simulink model "NeuromuscularModel_3R60CMG_3D"  (R2019b)
settings: Solver=ode15s  StartTime=0.0  StopTime=20  MaxStep=.001  MinStep=1e-34  RelTol=1e-5  AbsTol=1e-7  EnableMultiTasking=on
values from neighbouring files (symbols this model uses):
  animFrameRate = 30    [demorun.m]    (also in evaluateCost.m; optimize.m; optimizeCMG.m)
  dt_visual = 1/1000    (= 0.001)    [demorun.m]    (also in evaluateCost.m; optimize.m = 0.0333333333333; optimizeCMG.m)
  initialTargetAngle = 70*pi/180    (= 1.2217304764)    [setInit.m]
  LPreStimBFSHinit = initConditionsSagittal(12)    [assignInit.m]
  LPreStimGASinit = initConditionsSagittal(13)    [assignInit.m]
  LPreStimGLUinit = initConditionsSagittal(8)    [assignInit.m]
  LPreStimHABinit = initConditionsCoronal(6)    [assignInit.m]
  LPreStimHADinit = initConditionsCoronal(7)    [assignInit.m]
  LPreStimHAMinit = initConditionsSagittal(9)    [assignInit.m]
  LPreStimHFLinit = initConditionsSagittal(7)    [assignInit.m]
  LPreStimRFinit = initConditionsSagittal(10)    [assignInit.m]
  LPreStimSOLinit = initConditionsSagittal(14)    [assignInit.m]
  LPreStimTAinit = initConditionsSagittal(15)    [assignInit.m]
  LPreStimVASinit = initConditionsSagittal(11)    [assignInit.m]
  LTargetAngleInit = initConditionsSagittal(6)    [assignInit.m]
  LTargetAngleRInit = initConditionsCoronal(5)    [assignInit.m]
  RPreStimGLUinit = initConditionsSagittal(18)    [assignInit.m]
  RPreStimHABinit = initConditionsCoronal(9)    [assignInit.m]
  RPreStimHADinit = initConditionsCoronal(10)    [assignInit.m]
  RPreStimHAMinit = initConditionsSagittal(19)    [assignInit.m]
  RPreStimHFLinit = initConditionsSagittal(17)    [assignInit.m]
  RPreStimRFinit = initConditionsSagittal(20)    [assignInit.m]
  RTargetAngleInit = initConditionsSagittal(16)    [assignInit.m]
  RTargetAngleRInit = initConditionsCoronal(8)    [assignInit.m]
undefined symbols (not defined in the file or in its folder): DiscIntNeverNeededParam, g, hatLeftHipToCenterDistWidth, LongDelay, LongLoopDelay, MidDelay, ShortDelay, termination_height, thetaHATref, X, Y, Z
libraries: NeuroMuscularLibrary x96, nesl_utility x22, sm_lib x21, CMGlibrary x6, simulink x3
(part 3 of 3)

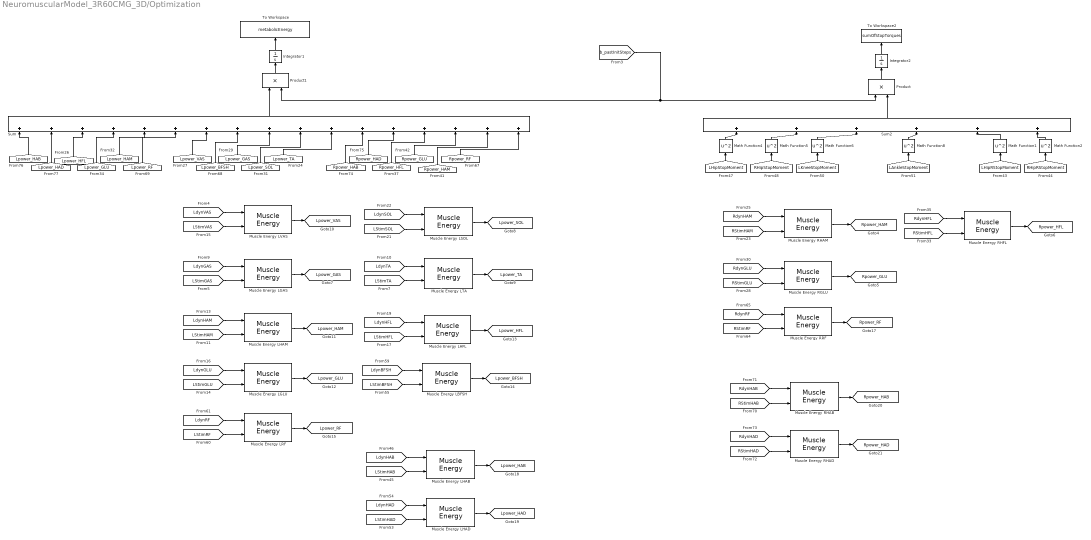
== system NeuromuscularModel_3R60CMG_3D/Optimization ==
  Integrator1 : Integrator
  Integrator2 : Integrator
  Math Function{1..2,4..6,8} (6 alike) : Math  Operator=square  SaturateOnIntegerOverflow=on
  Muscle Energy LBFSH : NeuroMuscularLibrary/Muscle Energy  lopt=loptBFSH  FT=FT_BFSH  Fmax=FmaxBFSH  vmax=vmaxBFSH
  Muscle Energy LGAS : NeuroMuscularLibrary/Muscle Energy  lopt=loptGAS  FT=FT_GAS  Fmax=FmaxGAS  vmax=vmaxGAS
  Muscle Energy LGLU : NeuroMuscularLibrary/Muscle Energy  lopt=loptGLU  FT=FT_GLU  Fmax=FmaxGLU  vmax=vmaxGLU
  Muscle Energy LHAB : NeuroMuscularLibrary/Muscle Energy  lopt=loptHAB  FT=FT_HAB  Fmax=FmaxHAB  vmax=vmaxHAB
  Muscle Energy LHAD : NeuroMuscularLibrary/Muscle Energy  lopt=loptHAD  FT=FT_HAD  Fmax=FmaxHAD  vmax=vmaxHAD
  Muscle Energy LHAM : NeuroMuscularLibrary/Muscle Energy  lopt=loptHAM  FT=FT_HAM  Fmax=FmaxHAM  vmax=vmaxHAM
  Muscle Energy LHFL : NeuroMuscularLibrary/Muscle Energy  lopt=loptHFL  FT=FT_HFL  Fmax=FmaxHFL  vmax=vmaxHFL
  Muscle Energy LRF : NeuroMuscularLibrary/Muscle Energy  lopt=loptRF  FT=FT_RF  Fmax=FmaxRF  vmax=vmaxRF
  Muscle Energy LSOL : NeuroMuscularLibrary/Muscle Energy  lopt=loptSOL  FT=FT_SOL  Fmax=FmaxSOL  vmax=vmaxSOL
  Muscle Energy LTA : NeuroMuscularLibrary/Muscle Energy  lopt=loptTA  FT=FT_TA  Fmax=FmaxTA  vmax=vmaxTA
  Muscle Energy LVAS : NeuroMuscularLibrary/Muscle Energy  lopt=loptVAS  FT=FT_VAS  Fmax=FmaxVAS  vmax=vmaxVAS
  Muscle Energy RGLU : NeuroMuscularLibrary/Muscle Energy  lopt=loptGLUamp  FT=FT_GLUamp  Fmax=FmaxGLUamp  vmax=vmaxGLUamp
  Muscle Energy RHAB : NeuroMuscularLibrary/Muscle Energy  lopt=loptHABamp  FT=FT_HABamp  Fmax=FmaxHABamp  vmax=vmaxHABamp
  Muscle Energy RHAD : NeuroMuscularLibrary/Muscle Energy  lopt=loptHADamp  FT=FT_HADamp  Fmax=FmaxHADamp  vmax=vmaxHADamp
  Muscle Energy RHAM : NeuroMuscularLibrary/Muscle Energy  lopt=loptHAMamp  FT=FT_HAMamp  Fmax=FmaxHAMamp  vmax=vmaxHAMamp
  Muscle Energy RHFL : NeuroMuscularLibrary/Muscle Energy  lopt=loptHFLamp  FT=FT_HFLamp  Fmax=FmaxHFLamp  vmax=vmaxHFLamp
  Muscle Energy RRF : NeuroMuscularLibrary/Muscle Energy  lopt=loptRFamp  FT=FT_RFamp  Fmax=FmaxRFamp  vmax=vmaxRFamp
  Product : Product
  Product1 : Product
  Sum : Sum  Inputs=+++++++++++++++++
  Sum2 : Sum  Inputs=++++++
  To Workspace : ToWorkspace  VariableName=metabolicEnergy  SampleTime=-1
      settings: MaxDataPoints=1
  To Workspace2 : ToWorkspace  VariableName=sumOfStopTorques  SampleTime=-1
      settings: MaxDataPoints=1
  tag scope: Lpower_BFSH=global, Lpower_GAS=global, Lpower_GLU=global, Lpower_HAB=global, Lpower_HAD=global, Lpower_HAM=global, Lpower_HFL=global, Lpower_RF=global, Lpower_SOL=global, Lpower_TA=global, Lpower_VAS=global, Rpower_GLU=global, Rpower_HAB=global, Rpower_HAD=global, Rpower_HAM=global, Rpower_HFL=global, Rpower_RF=global
  wires:
  [RdynHAM] -> Muscle Energy RHAM/1
  [RStimHAM] -> Muscle Energy RHAM/2
  [RdynGLU] -> Muscle Energy RGLU/1
  [RStimGLU] -> Muscle Energy RGLU/2
  [RdynHFL] -> Muscle Energy RHFL/1
  [RStimHFL] -> Muscle Energy RHFL/2
  Muscle Energy RHAM/1 -> [Rpower_HAM]
  Muscle Energy RGLU/1 -> [Rpower_GLU]
  Muscle Energy RHFL/1 -> [Rpower_HFL]
  [Lpower_HAB] -> Sum/1
  [Lpower_VAS] -> Sum/7
  [Lpower_RF] -> Sum/6
  [Lpower_HAM] -> Sum/5
  [Lpower_GLU] -> Sum/4
  [Lpower_HFL] -> Sum/3
  [Lpower_HAD] -> Sum/2
  [LdynSOL] -> Muscle Energy LSOL/1
  [LStimSOL] -> Muscle Energy LSOL/2
  [LStimVAS] -> Muscle Energy LVAS/2
  [LStimGAS] -> Muscle Energy LGAS/2
  Muscle Energy LVAS/1 -> [Lpower_VAS]
  Muscle Energy LGAS/1 -> [Lpower_GAS]
  Muscle Energy LSOL/1 -> [Lpower_SOL]
  Muscle Energy LTA/1 -> [Lpower_TA]
  [LdynTA] -> Muscle Energy LTA/1
  [LStimTA] -> Muscle Energy LTA/2
  [LdynHAM] -> Muscle Energy LHAM/1
  [LStimHAM] -> Muscle Energy LHAM/2
  [LdynGLU] -> Muscle Energy LGLU/1
  [LStimGLU] -> Muscle Energy LGLU/2
  [LdynHFL] -> Muscle Energy LHFL/1
  [LStimHFL] -> Muscle Energy LHFL/2
  Muscle Energy LHAM/1 -> [Lpower_HAM]
  Muscle Energy LGLU/1 -> [Lpower_GLU]
  Muscle Energy LHFL/1 -> [Lpower_HFL]
  [LdynGAS] -> Muscle Energy LGAS/1
  [LdynVAS] -> Muscle Energy LVAS/1
  [Lpower_SOL] -> Sum/10
  [Rpower_HAM] -> Sum/16
  [Rpower_GLU] -> Sum/15
  [Rpower_HFL] -> Sum/14
  [Rpower_HAD] -> Sum/13
  [Rpower_HAB] -> Sum/12
  [Lpower_TA] -> Sum/11
  Integrator1/1 -> To Workspace/1
  Sum/1 -> Product1/1
  Integrator2/1 -> To Workspace2/1
  Math Function4/1 -> Sum2/1
  [LHipStopMoment] -> Math Function4/1
  Math Function5/1 -> Sum2/2
  [RHipStopMoment] -> Math Function5/1
  Math Function6/1 -> Sum2/3
  [LKneeStopMoment] -> Math Function6/1
  [LAnkleStopMoment] -> Math Function8/1
  Math Function8/1 -> Sum2/4
  Product/1 -> Integrator2/1
  Sum2/1 -> Product/2
  Product1/1 -> Integrator1/1
  Muscle Energy LBFSH/1 -> [Lpower_BFSH]
  [LStimBFSH] -> Muscle Energy LBFSH/2
  [LdynBFSH] -> Muscle Energy LBFSH/1
  [LdynRF] -> Muscle Energy LRF/1
  [LStimRF] -> Muscle Energy LRF/2
  Muscle Energy LRF/1 -> [Lpower_RF]
  Muscle Energy RRF/1 -> [Rpower_RF]
  [RdynRF] -> Muscle Energy RRF/1
  [RStimRF] -> Muscle Energy RRF/2
  [Lpower_BFSH] -> Sum/8
  [Lpower_GAS] -> Sum/9
  [Rpower_RF] -> Sum/17
  Math Function1/1 -> Sum2/5
  [LHipRStopMoment] -> Math Function1/1
  [RHipRStopMoment] -> Math Function2/1
  Muscle Energy LHAB/1 -> [Lpower_HAB]
  [LStimHAB] -> Muscle Energy LHAB/2
  [LdynHAB] -> Muscle Energy LHAB/1
  [LdynHAD] -> Muscle Energy LHAD/1
  [LStimHAD] -> Muscle Energy LHAD/2
  Muscle Energy LHAD/1 -> [Lpower_HAD]
  Muscle Energy RHAD/1 -> [Rpower_HAD]
  [RStimHAD] -> Muscle Energy RHAD/2
  [RdynHAD] -> Muscle Energy RHAD/1
  [RdynHAB] -> Muscle Energy RHAB/1
  [RStimHAB] -> Muscle Energy RHAB/2
  Muscle Energy RHAB/1 -> [Rpower_HAB]
  Math Function2/1 -> Sum2/6
  [b_pastInitSteps] -> Product1/2, Product/1

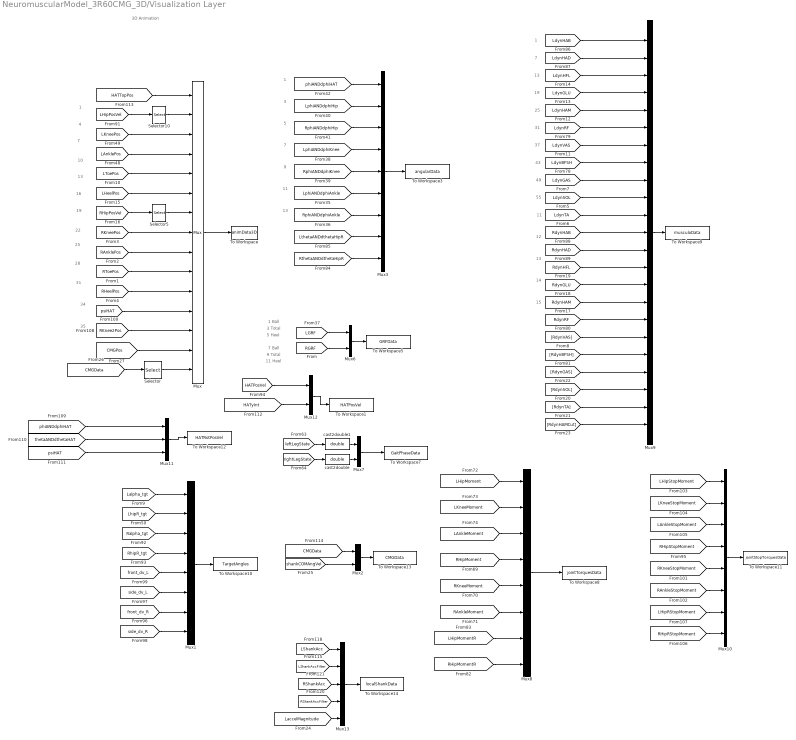
== system NeuromuscularModel_3R60CMG_3D/Visualization Layer ==
  note: 31
  note: 28
  note: 25
  note: 22
  note: 19
  note: 16
  note: 13
  note: 10
  note: 7
  note: 4
  note: 1
  note: 3D Animation
  note: 1
  note: 13
  note: 3
  note: 5
  note: 7
  note: 9
  note: 11
  note: 9 Total
  note: 1 Ball
  note: 5 Heel
  note: 11 Heel
  note: 3 Total
  note: 7 Ball
  note: 7
  note: 12
  note: 13
  note: 55
  note: 14
  note: 19
  note: 1
  note: 43
  note: 49
  note: 37
  note: 25
  note: 11
  note: 13
  note: 15
  note: 31
  note: 34
  note: 35
  Mux : Mux  Inputs=15
  Mux1 : Mux  Inputs=8
  Mux10 : Mux  Inputs=8
  Mux11 : Mux  Inputs=3
  Mux{2,6..7,12} (4 alike) : Mux  Inputs=2
  Mux13 : Mux  Inputs=5
  Mux3 : Mux  Inputs=9
  Mux8 : Mux  Inputs=8
  Mux9 : Mux  Inputs=23
  Selector : Selector  InputPortWidth=17  IndexOptions=Index vector (dialog)  Indices=[1]  OutputSizes=1
  Selector10 : Selector  InputPortWidth=6  IndexOptions=Index vector (dialog)  Indices=[1 2 3]  OutputSizes=1
  Selector5 : Selector  InputPortWidth=6  IndexOptions=Index vector (dialog)  Indices=[1 2 3]  OutputSizes=1
  To Workspace : ToWorkspace  VariableName=animData3D  SaveFormat=Structure With Time  SampleTime=1/animFrameRate
  To Workspace1 : ToWorkspace  VariableName=HATPosVel  SaveFormat=Structure With Time  SampleTime=dt_visual
  To Workspace10 : ToWorkspace  VariableName=TargetAngles  SaveFormat=Structure With Time  SampleTime=dt_visual
  To Workspace11 : ToWorkspace  VariableName=jointStopTorquesData  SaveFormat=Structure With Time  SampleTime=dt_visual
  To Workspace12 : ToWorkspace  VariableName=HATRotPosVel  SaveFormat=Structure With Time  SampleTime=dt_visual
  To Workspace13 : ToWorkspace  VariableName=CMGData  SaveFormat=Structure With Time  SampleTime=dt_visual
  To Workspace14 : ToWorkspace  VariableName=localShankData  SaveFormat=Structure With Time  SampleTime=dt_visual
  To Workspace3 : ToWorkspace  VariableName=angularData  SaveFormat=Structure With Time  SampleTime=dt_visual
  To Workspace5 : ToWorkspace  VariableName=GRFData  SaveFormat=Structure With Time  SampleTime=dt_visual
  To Workspace7 : ToWorkspace  VariableName=GaitPhaseData  SaveFormat=Structure With Time  SampleTime=dt_visual
  To Workspace8 : ToWorkspace  VariableName=jointTorquesData  SaveFormat=Structure With Time  SampleTime=dt_visual
  To Workspace9 : ToWorkspace  VariableName=musculoData  SaveFormat=Structure With Time  SampleTime=dt_visual
  cast2double : DataTypeConversion  OutDataTypeStr=double
  cast2double1 : DataTypeConversion  OutDataTypeStr=double
  wires:
  [RphiANDdphiAnkle] -> Mux3/7
  Mux6/1 -> To Workspace5/1
  [RGRF] -> Mux6/2
  [phiANDdphiHAT] -> Mux3/1
  Mux3/1 -> To Workspace3/1
  [LphiANDdphiAnkle] -> Mux3/6
  [LphiANDdphiKnee] -> Mux3/4
  [LGRF] -> Mux6/1
  [LphiANDdphiHip] -> Mux3/2
  [RphiANDdphiKnee] -> Mux3/5
  [RphiANDdphiHip] -> Mux3/3
  [rightLegState] -> cast2double/1
  Mux7/1 -> To Workspace7/1
  [leftLegState] -> cast2double1/1
  Mux8/1 -> To Workspace8/1
  [LHipMoment] -> Mux8/1
  [LKneeMoment] -> Mux8/2
  [LAnkleMoment] -> Mux8/3
  [RHipMoment] -> Mux8/4
  [RKneeMoment] -> Mux8/5
  [RAnkleMoment] -> Mux8/6
  Mux9/1 -> To Workspace9/1
  [RdynHAM] -> Mux9/16
  [LdynHFL] -> Mux9/3
  [RdynGLU] -> Mux9/15
  [RdynVAS] -> Mux9/18
  [LdynBFSH] -> Mux9/8
  [RdynGAS] -> Mux9/20
  [RdynBFSH] -> Mux9/19
  [LdynVAS] -> Mux9/7
  [LdynGAS] -> Mux9/9
  [LdynSOL] -> Mux9/10
  [LdynRF] -> Mux9/6
  [LdynHAM] -> Mux9/5
  [LdynGLU] -> Mux9/4
  [LdynTA] -> Mux9/11
  [RdynRF] -> Mux9/17
  [RdynHFL] -> Mux9/14
  [RdynSOL] -> Mux9/21
  [RdynTA] -> Mux9/22
  [RdynHAMCut] -> Mux9/23
  [LHipMomentR] -> Mux8/7
  [RHipMomentR] -> Mux8/8
  [LthetaANDdthetaHipR] -> Mux3/8
  [RthetaANDdthetaHipR] -> Mux3/9
  [RdynHAB] -> Mux9/12
  [RdynHAD] -> Mux9/13
  [LdynHAB] -> Mux9/1
  [LdynHAD] -> Mux9/2
  Selector5/1 -> Mux/7
  [LAnklePos] -> Mux/4
  [LKneePos] -> Mux/3
  [LHeelPos] -> Mux/6
  [LToePos] -> Mux/5
  [RToePos] -> Mux/10
  [LHipPosVel] -> Selector10/1
  Mux/1 -> To Workspace/1
  [RAnklePos] -> Mux/9
  [RHipPosVel] -> Selector5/1
  Selector10/1 -> Mux/2
  [RHeelPos] -> Mux/11
  [RKneePos] -> Mux/8
  [Lalpha_tgt] -> Mux1/1
  [front_dv_R] -> Mux1/7
  [side_dv_L] -> Mux1/6
  [side_dv_R] -> Mux1/8
  [RhipR_tgt] -> Mux1/4
  Mux1/1 -> To Workspace10/1
  [front_dv_L] -> Mux1/5
  [HATPosVel] -> Mux12/1
  [LhipR_tgt] -> Mux1/2
  Mux11/1 -> To Workspace12/1
  [Ralpha_tgt] -> Mux1/3
  [LAnkleStopMoment] -> Mux10/3
  Mux10/1 -> To Workspace11/1
  [LHipStopMoment] -> Mux10/1
  [LKneeStopMoment] -> Mux10/2
  [RAnkleStopMoment] -> Mux10/6
  [RHipStopMoment] -> Mux10/4
  [LHipRStopMoment] -> Mux10/7
  [RKneeStopMoment] -> Mux10/5
  [RHipRStopMoment] -> Mux10/8
  [RKnee2Pos] -> Mux/13
  [thetaANDdthetaHAT] -> Mux11/2
  [psiHAT] -> Mux11/3
  [phiANDdphiHAT] -> Mux11/1
  [psiHAT] -> Mux/12
  Mux12/1 -> To Workspace1/1
  [HATyInt] -> Mux12/2
  [HATTopPos] -> Mux/1
  cast2double1/1 -> Mux7/1
  cast2double/1 -> Mux7/2
  [LaccelMagnitude] -> Mux13/5
  [LShankAccFilter] -> Mux13/2
  Mux13/1 -> To Workspace14/1
  [CMGData] -> Mux2/1
  [LShankAcc] -> Mux13/1
  [RShankAcc] -> Mux13/3
  [RShankAccFilter] -> Mux13/4
  [shankCOMAngVel] -> Mux2/2
  Mux2/1 -> To Workspace13/1
  Selector/1 -> Mux/15
  [CMGData] -> Selector/1
  [CMGPos] -> Mux/14

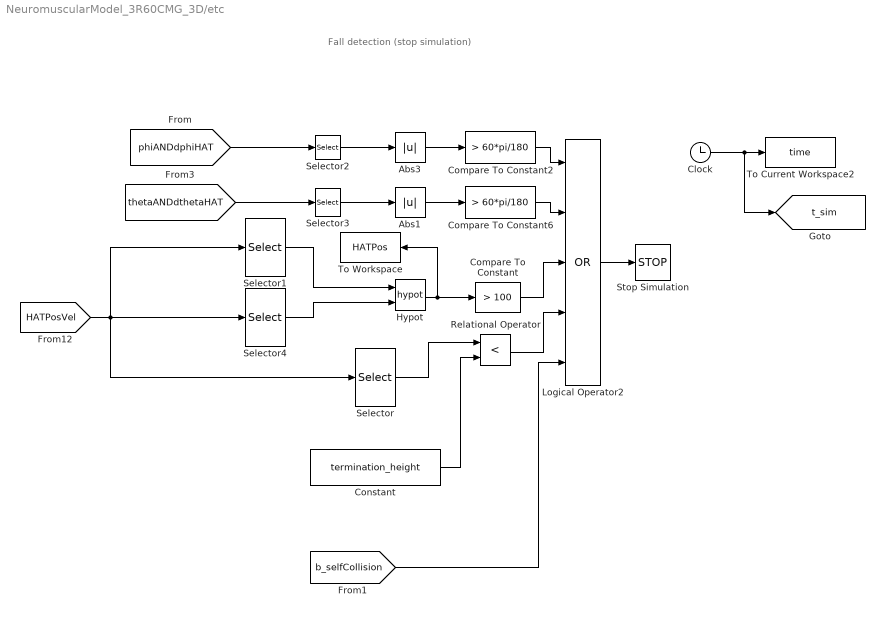
== system NeuromuscularModel_3R60CMG_3D/etc ==
  note: Fall detection
      | (stop simulation)
  Abs1 : Abs
  Abs3 : Abs
  Clock : Clock
  Compare To Constant : simulink/Logic and Bit Operations/Compare To Constant  relop=>  const=100  OutDataTypeStr=boolean
  Compare To Constant2 : simulink/Logic and Bit Operations/Compare To Constant  relop=>  const=60*pi/180  OutDataTypeStr=boolean
  Compare To Constant6 : simulink/Logic and Bit Operations/Compare To Constant  relop=>  const=60*pi/180  OutDataTypeStr=boolean
  Constant : Constant  Value=termination_height
  Hypot : Math  Operator=hypot  SignedPower=off  SaturateOnIntegerOverflow=on
  Logical Operator2 : Logic  Operator=OR  Inputs=5  AllPortsSameDT=off  OutDataTypeStr=boolean
  Relational Operator : RelationalOperator  Operator=<  OutDataTypeStr=boolean  RndMeth=Nearest
  Selector : Selector  InputPortWidth=6  IndexOptions=Index vector (dialog)  Indices=[3]  OutputSizes=1
  Selector1 : Selector  InputPortWidth=6  IndexOptions=Index vector (dialog)  Indices=[1]  OutputSizes=1
  Selector2 : Selector  InputPortWidth=2  IndexOptions=Index vector (dialog)  Indices=[1]  OutputSizes=1
  Selector3 : Selector  InputPortWidth=2  IndexOptions=Index vector (dialog)  Indices=[1]  OutputSizes=1
  Selector4 : Selector  InputPortWidth=6  IndexOptions=Index vector (dialog)  Indices=[2]  OutputSizes=1
  Stop Simulation : Stop
  To Current Workspace2 : ToWorkspace  VariableName=time  SampleTime=-1
      settings: MaxDataPoints=1
  To Workspace : ToWorkspace  VariableName=HATPos  SampleTime=-1
      settings: MaxDataPoints=1
  tag scope: t_sim=global
  wires:
  Selector2/1 -> Abs3/1
  Abs3/1 -> Compare To Constant2/1
  Compare To Constant2/1 -> Logical Operator2/1
  Logical Operator2/1 -> Stop Simulation/1
  Selector3/1 -> Abs1/1
  Abs1/1 -> Compare To Constant6/1
  Compare To Constant6/1 -> Logical Operator2/2
  Compare To Constant/1 -> Logical Operator2/3
  Selector/1 -> Relational Operator/1
  Constant/1 -> Relational Operator/2
  Relational Operator/1 -> Logical Operator2/4
  Clock/1 -> [t_sim], To Current Workspace2/1
  [phiANDdphiHAT] -> Selector2/1
  [thetaANDdthetaHAT] -> Selector3/1
  Selector1/1 -> Hypot/1
  Hypot/1 -> To Workspace/1, Compare To Constant/1
  [HATPosVel] -> Selector1/1, Selector/1, Selector4/1
  Selector4/1 -> Hypot/2
  [b_selfCollision] -> Logical Operator2/5

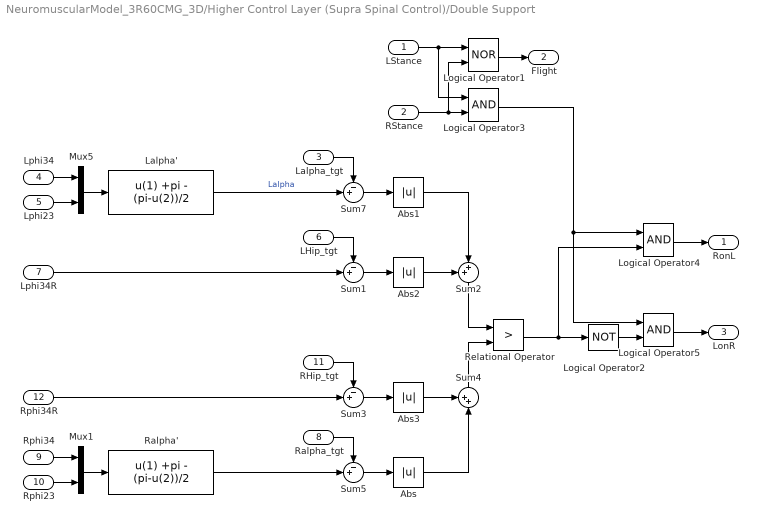
== system NeuromuscularModel_3R60CMG_3D/Higher Control Layer (Supra Spinal Control)/Double Support ==
  LStance : Inport
  RStance : Inport  Port=2
  Lalpha_tgt : Inport  Port=3
  Lphi34 : Inport  Port=4
  Lphi23 : Inport  Port=5
  LHip_tgt : Inport  Port=6
  Lphi34R : Inport  Port=7
  Ralpha_tgt : Inport  Port=8
  Rphi34 : Inport  Port=9
  Rphi23 : Inport  Port=10
  RHip_tgt : Inport  Port=11
  Rphi34R : Inport  Port=12
  Abs{,1..3} (4 alike) : Abs  ZeroCross=off
  Lalpha' : Fcn  Expr=u(1) +pi - (pi-u(2))/2
  Logical Operator1 : Logic  Operator=NOR  AllPortsSameDT=off  OutDataTypeStr=boolean
  Logical Operator2 : Logic  Operator=NOT  AllPortsSameDT=off
  Logical Operator3 : Logic  AllPortsSameDT=off
  Logical Operator4 : Logic  AllPortsSameDT=off
  Logical Operator5 : Logic  AllPortsSameDT=off
  Mux1 : Mux  Inputs=2
  Mux5 : Mux  Inputs=2
  Ralpha' : Fcn  Expr=u(1) +pi - (pi-u(2))/2
  Relational Operator : RelationalOperator  Operator=>  ZeroCross=off  RndMeth=Nearest
  Sum{1,3,5,7} (4 alike) : Sum  Inputs=-+|
  Sum2 : Sum  Inputs=++|
  Sum4 : Sum  Inputs=++|
  RonL : Outport
  Flight : Outport  Port=2
  LonR : Outport  Port=3
  wires:
  Lalpha'/1 -> Sum7/2  "Lalpha"
  Mux5/1 -> Lalpha'/1
  Ralpha'/1 -> Sum5/2
  Mux1/1 -> Ralpha'/1
  Sum5/1 -> Abs/1
  Sum7/1 -> Abs1/1
  LStance/1 -> Logical Operator3/1, Logical Operator1/1
  RStance/1 -> Logical Operator3/2, Logical Operator1/2
  Lalpha_tgt/1 -> Sum7/1
  Lphi34/1 -> Mux5/1
  Lphi23/1 -> Mux5/2
  Ralpha_tgt/1 -> Sum5/1
  Rphi34/1 -> Mux1/1
  Rphi23/1 -> Mux1/2
  Logical Operator1/1 -> Flight/1
  LHip_tgt/1 -> Sum1/1
  Lphi34R/1 -> Sum1/2
  Sum1/1 -> Abs2/1
  Abs2/1 -> Sum2/1
  Abs1/1 -> Sum2/2
  Sum2/1 -> Relational Operator/1
  RHip_tgt/1 -> Sum3/1
  Rphi34R/1 -> Sum3/2
  Sum3/1 -> Abs3/1
  Abs/1 -> Sum4/2
  Abs3/1 -> Sum4/1
  Sum4/1 -> Relational Operator/2
  Logical Operator4/1 -> RonL/1
  Logical Operator2/1 -> Logical Operator5/2
  Logical Operator5/1 -> LonR/1
  Relational Operator/1 -> Logical Operator2/1, Logical Operator4/2
  Logical Operator3/1 -> Logical Operator5/1, Logical Operator4/1
